simulink model "dpr_sim"  (R2020b)
settings: Solver=FixedStepDiscrete  StartTime=0.0  StopTime=stopTime  RelTol=1e-3
InitFcn:
  | initCallback
StopFcn:
  | stopCallback
undefined symbols (not defined in the file or in its folder): config
libraries: dspsrcs4 x1, hdlsllib x1
settings Model: SimulationMode=accelerator  Creator=Ross  LastModifiedBy=tyler
settings SolverCC: AutoInsertRateTranBlk=on
settings DataIOCC: ReturnWorkspaceOutputs=off
settings OptimizationCC: BlockReduction=off  ConditionallyExecuteInputs=off  DefaultParameterBehavior=Inlined
settings DebuggingCC: SignalInfNanChecking=error  SignalRangeChecking=warning  ReadBeforeWriteMsg=DisableAll  WriteAfterWriteMsg=DisableAll  WriteAfterReadMsg=DisableAll  AlgebraicLoopMsg=error  MultiTaskDSMMsg=none  SingleTaskRateTransMsg=error  ParameterUnderflowMsg=warning  UnderSpecifiedDataTypeMsg=error  PregeneratedLibrarySubsystemCodeDiagnostic=none  ArithmeticOperatorsInVariantConditions=warning
settings HardwareCC: ProdBitPerPointer=32  ProdBitPerSizeT=32  ProdBitPerPtrDiffT=32  ProdLargestAtomicFloat=None  ProdIntDivRoundTo=Undefined  ProdEndianess=Unspecified  ProdWordSize=32  ProdHWDeviceType=ASIC/FPGA->ASIC/FPGA  TargetBitPerPointer=64  TargetBitPerSizeT=64  TargetBitPerPtrDiffT=64  TargetLongLongMode=on  TargetIntDivRoundTo=Zero  TargetEndianess=LittleEndian  TargetWordSize=64  TargetHWDeviceType=Custom Processor->MATLAB Host Computer  ProdEqTarget=off
settings ModelReferenceCC: UpdateModelReferenceTargets=IfOutOfDate
settings SFSimCC: SFSimEcho=off  SimUseLocalCustomCode=off  CustomCodeUndefinedFunction=UseInterfaceOnly
settings RTWCC: RTWUseLocalCustomCode=off

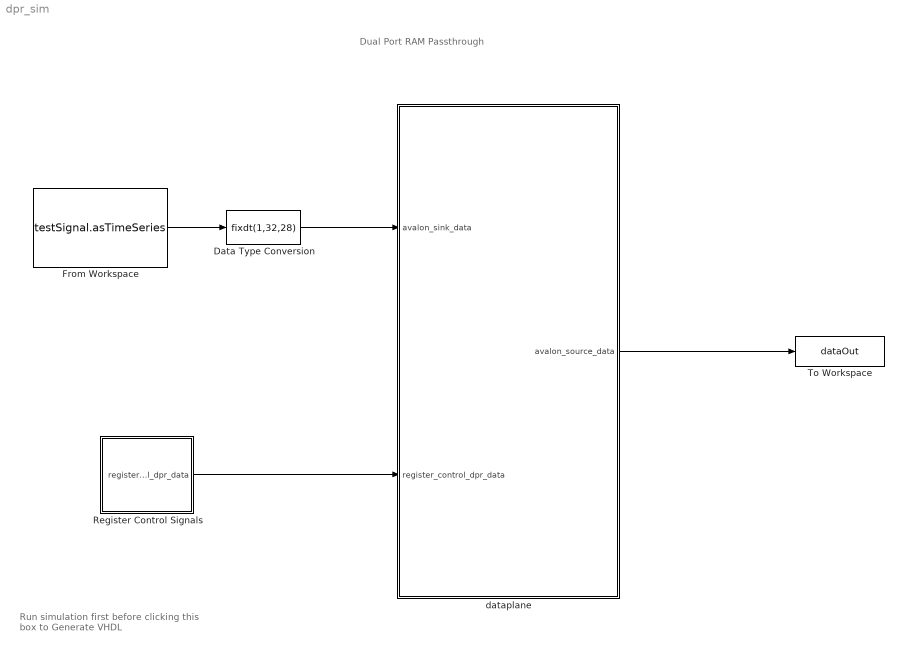
== system dpr_sim ==
  note: Dual Port RAM Passthrough
  note: Run simulation first
      | before clicking this box to
      | Generate VHDL
  Data Type Conversion : DataTypeConversion  OutDataTypeStr=fixdt(1,32,28)
  From Workspace : FromWorkspace  VariableName=testSignal.asTimeSeries  OutDataTypeStr=double  SampleTime=1 / config.system.sampleClockFrequency  Interpolate=off  OutputAfterFinalValue=Setting to zero
  Register Control Signals : Subsystem
  To Workspace : ToWorkspace  VariableName=dataOut  SaveFormat=Timeseries  SampleTime=-1
      settings: Save2DSignal=2-D array (concatenate along first dimension)
  dataplane : Subsystem  TreatAsAtomicUnit=on
  wires:
  dataplane/1(avalon_source_data) -> To Workspace/1
  From Workspace/1 -> Data Type Conversion/1
  Data Type Conversion/1 -> dataplane/1(avalon_sink_data)
  Register Control Signals/1("register_control_dpr_data ") -> dataplane/2(register_control_dpr_data)

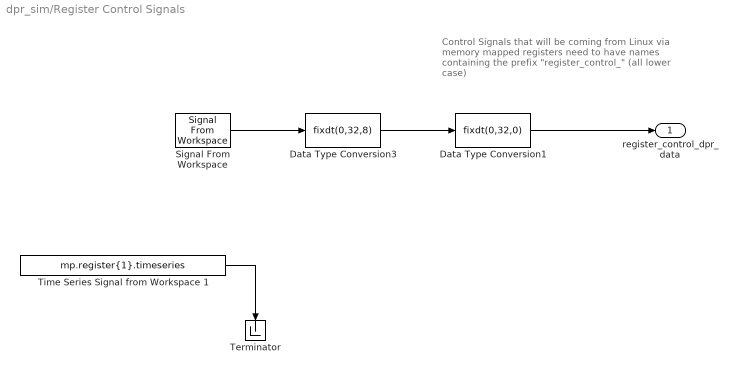
== system dpr_sim/Register Control Signals ==
  note: Control Signals that will be coming from Linux via
      | memory mapped registers need to have names
      | containing the prefix "register_control_"
      | (all lower case)
  Data Type Conversion1 : DataTypeConversion  OutDataTypeStr=fixdt(0,32,0)  ConvertRealWorld=Stored Integer (SI)
  Data Type Conversion3 : DataTypeConversion  OutDataTypeStr=fixdt(0,32,8)  ConvertRealWorld=Stored Integer (SI)
  Signal From Workspace : dspsrcs4/Signal From Workspace  X=dprDataIn  Ts=1 / config.system.sampleClockFrequency  nsamps=1  OutputAfterFinalValue=Holding final value  ignoreOrWarnInputAndFrameLengths=off  OutputFrames=off
  Terminator : Terminator
  Time Series Signal from Workspace 1 : FromWorkspace  VariableName=mp.register{1}.timeseries  OutDataTypeStr=double  SampleTime=1 / config.system.sampleClockFrequency
  "register_control_dpr_data " : Outport  VectorParamsAs1DForOutWhenUnconnected=off
  wires:
  Data Type Conversion3/1 -> Data Type Conversion1/1
  Data Type Conversion1/1 -> "register_control_dpr_data "/1
  Signal From Workspace/1 -> Data Type Conversion3/1
  Time Series Signal from Workspace 1/1 -> Terminator/1

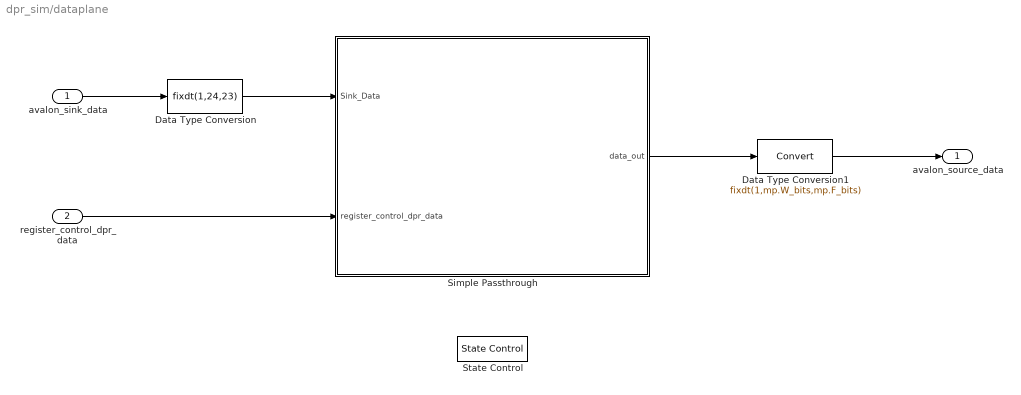
== system dpr_sim/dataplane ==
  avalon_sink_data : Inport
  register_control_dpr_data : Inport  Port=2
  Data Type Conversion : DataTypeConversion  OutDataTypeStr=fixdt(1,24,23)
  Data Type Conversion1 : DataTypeConversion  OutDataTypeStr=fixdt(1,mp.W_bits,mp.F_bits)
  "Simple Passthrough " : Subsystem
  State Control : StateControl  StateControl=Synchronous
  avalon_source_data : Outport  VectorParamsAs1DForOutWhenUnconnected=off
  wires:
  Data Type Conversion1/1 -> avalon_source_data/1
  avalon_sink_data/1 -> Data Type Conversion/1
  "Simple Passthrough "/1(data_out) -> Data Type Conversion1/1
  Data Type Conversion/1 -> "Simple Passthrough "/1(Sink_Data)
  register_control_dpr_data/1 -> "Simple Passthrough "/2(register_control_dpr_data)

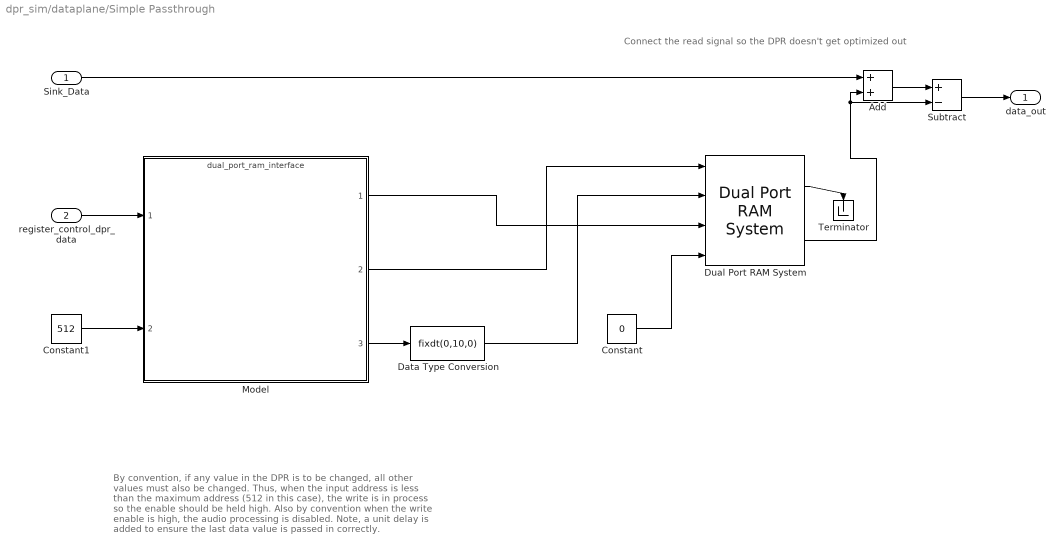
== system dpr_sim/dataplane/Simple Passthrough  ==
  note: Connect the read signal so the DPR doesn't get optimized out
  note: By convention, if any value in the DPR is to be changed, all other
      | values must also be changed.  Thus, when the input address is
      | less than the maximum address (512 in this case), the write is in
      | process so the enable should be held high.  Also by convention
      | when the write enable is high, the audio processing is disabled.
      | Note, a unit delay is added to ensure the last data value is passed
      | in correctly.
  Sink_Data : Inport
  register_control_dpr_data : Inport  Port=2
  Add : Sum
  Constant : Constant  Value=0  OutDataTypeStr=fixdt(0,10,0)  SampleTime=-1
  Constant1 : Constant  Value=512  OutDataTypeStr=uint32  SampleTime=-1
  Data Type Conversion : DataTypeConversion  OutDataTypeStr=fixdt(0,10,0)
  Dual Port RAM System : hdlsllib/HDL RAMs/Dual Port RAM System  RAMType=Dual port  WriteOutputValue=New data  RAMInitialValue=0  SimulateUsing=Code generation
      settings: SourceProductBaseCode=SL
  Model : ModelReference  ModelNameDialog=dual_port_ram_interface.slx  SimulationMode=Normal  ModelReferenceVersion=1.113
  Subtract : Sum  Inputs=+-
  Terminator : Terminator
  data_out : Outport
  wires:
  Model/2 -> Dual Port RAM System/1
  Constant/1 -> Dual Port RAM System/4
  Sink_Data/1 -> Add/1
  Add/1 -> Subtract/1
  Dual Port RAM System/2 -> Add/2, Subtract/2
  Subtract/1 -> data_out/1
  Dual Port RAM System/1 -> Terminator/1
  Model/1 -> Dual Port RAM System/3
  Model/3 -> Data Type Conversion/1
  Constant1/1 -> Model/2
  register_control_dpr_data/1 -> Model/1
  Data Type Conversion/1 -> Dual Port RAM System/2
